simulink model "RobustInvDyn"  (R2024b)
settings: Solver=ode15s  StartTime=0.0  StopTime=10  MinStep=0.0000001
InitFcn:
  | addpath('./../Robot Description/Robot Data Package/meshes/visual/')
  | addpath('./../Dynamics and Kinematics/')
  | 
  | % Controller Design
  | Design;
values from neighbouring files (symbols this model uses):
  alpha = 0.9    [Design.m]
  B = [zeros(n, n); eye(n)]    [Design.m]
  epsilon = 0.01    [Design.m]
  gamma1 = 3.5    [Design.m]
  gamma2 = 1.8    [Design.m]
  gamma3 = 5    [Design.m]
  Kd = 1000    [Design.m]
  Kp = 250000    [Design.m]
  P = lyap(A', Q)    [Design.m]
  qInitDM = [rand(n, 1); zeros(n, 1)]    [Design.m]
settings Model: Creator=Banaan  LastModifiedBy=Asus

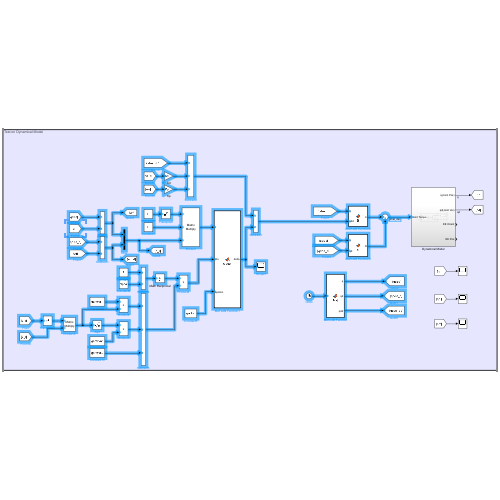
[thumbnail: Simulink's stored preview of the top-level diagram]
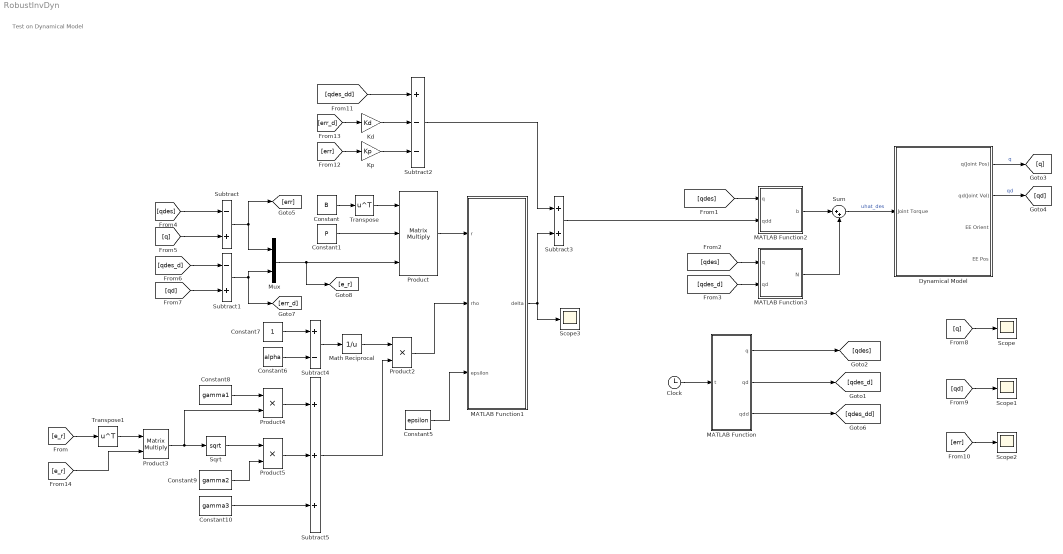
== system RobustInvDyn ==
  note: Test on Dynamical Model
  Clock : Clock
  Constant : Constant  Value=B
  Constant1 : Constant  Value=P
  Constant10 : Constant  Value=gamma3
  Constant5 : Constant  Value=epsilon
  Constant6 : Constant  Value=alpha
  Constant7 : Constant
  Constant8 : Constant  Value=gamma1
  Constant9 : Constant  Value=gamma2
  Dynamical Model : Subsystem
  Kd : Gain  Gain=Kd
  Kp : Gain  Gain=Kp
  MATLAB Function : MATLAB Function  TreatAsAtomicUnit=on
  MATLAB Function1 : MATLAB Function  TreatAsAtomicUnit=on
  MATLAB Function2 : MATLAB Function  TreatAsAtomicUnit=on
  MATLAB Function3 : MATLAB Function  TreatAsAtomicUnit=on
  Math Reciprocal : Math  Operator=reciprocal  SignedPower=on
  Mux : Mux  Inputs=2
  Product : Product  Inputs=3  Multiplication=Matrix(*)
  Product2 : Product
  Product3 : Product  Multiplication=Matrix(*)
  Product4 : Product
  Product5 : Product
  Scope{,1..3} (4 alike) : Scope
  Sqrt : Sqrt
  Subtract : Sum  Inputs=-+
  Subtract1 : Sum  Inputs=-+
  Subtract2 : Sum  Inputs=+--
  Subtract3 : Sum
  Subtract4 : Sum  Inputs=+-
  Subtract5 : Sum  Inputs=+++
  Sum : Sum  Inputs=|++
  Transpose : Math  Operator=transpose
  Transpose1 : Math  Operator=transpose
  wires:
  [qdes] -> MATLAB Function2/1(q)
  [qdes_d] -> MATLAB Function3/2(qd)
  [qdes] -> MATLAB Function3/1(q)
  MATLAB Function2/1(b) -> Sum/1
  MATLAB Function3/1(N) -> Sum/2
  Dynamical Model/1(q(Joint Pos)) -> [q]  "q"
  Dynamical Model/2(qd(Joint Vel)) -> [qd]  "qd"
  [q] -> Scope/1
  [qd] -> Scope1/1
  [err] -> Scope2/1
  MATLAB Function/3(qdd) -> [qdes_dd]
  MATLAB Function/2(qd) -> [qdes_d]
  Clock/1 -> MATLAB Function/1(t)
  MATLAB Function/1(q) -> [qdes]
  [qdes] -> Subtract/1
  [q] -> Subtract/2
  [qdes_d] -> Subtract1/1
  [qd] -> Subtract1/2
  Sum/1 -> Dynamical Model/1(Joint Torque)  "uhat_des"
  [qdes_dd] -> Subtract2/1
  Kd/1 -> Subtract2/2
  Kp/1 -> Subtract2/3
  Subtract/1 -> [err], Mux/1
  Subtract1/1 -> [err_d], Mux/2
  Constant/1 -> Transpose/1
  Transpose/1 -> Product/1
  Constant1/1 -> Product/2
  Mux/1 -> [e_r], Product/3
  Product/1 -> MATLAB Function1/1(r)
  [err] -> Kp/1
  [err_d] -> Kd/1
  MATLAB Function1/1(delta) -> Scope3/1, Subtract3/2
  Subtract2/1 -> Subtract3/1
  Subtract3/1 -> MATLAB Function2/2(qdd)
  Constant5/1 -> MATLAB Function1/3(epsilon)
  Constant7/1 -> Subtract4/1
  Constant6/1 -> Subtract4/2
  Subtract4/1 -> Math Reciprocal/1
  Math Reciprocal/1 -> Product2/1
  Subtract5/1 -> Product2/2
  Product2/1 -> MATLAB Function1/2(rho)
  [e_r] -> Transpose1/1
  Transpose1/1 -> Product3/1
  [e_r] -> Product3/2
  Constant8/1 -> Product4/1
  Product3/1 -> Product4/2, Sqrt/1
  Sqrt/1 -> Product5/1
  Constant9/1 -> Product5/2
  Product4/1 -> Subtract5/1
  Product5/1 -> Subtract5/2
  Constant10/1 -> Subtract5/3

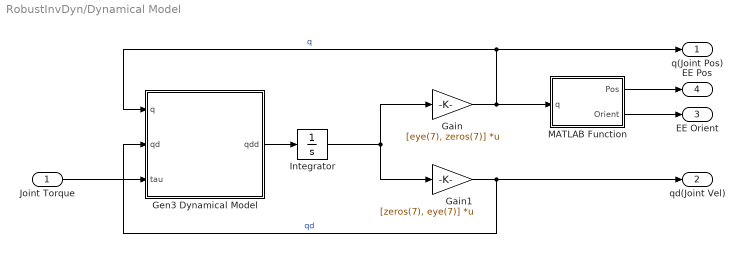
== system RobustInvDyn/Dynamical Model ==
  Joint Torque : Inport
  Gain : Gain  Gain=[eye(7), zeros(7)]  Multiplication=Matrix(K*u)
  Gain1 : Gain  Gain=[zeros(7), eye(7)]  Multiplication=Matrix(K*u)
  Gen3 Dynamical Model : MATLAB Function  TreatAsAtomicUnit=on
  Integrator : Integrator  InitialCondition=qInitDM
  MATLAB Function : MATLAB Function  TreatAsAtomicUnit=on
  q(Joint Pos) : Outport
  qd(Joint Vel) : Outport  Port=2
  EE Orient : Outport  Port=3
  EE Pos : Outport  Port=4
  wires:
  Integrator/1 -> Gain/1, Gain1/1
  Gain/1 -> MATLAB Function/1(q), Gen3 Dynamical Model/1(q), q(Joint Pos)/1  "q"
  Gen3 Dynamical Model/1(qdd) -> Integrator/1
  Gain1/1 -> qd(Joint Vel)/1, Gen3 Dynamical Model/2(qd)  "qd"
  Joint Torque/1 -> Gen3 Dynamical Model/3(tau)
  MATLAB Function/1(Pos) -> EE Pos/1
  MATLAB Function/2(Orient) -> EE Orient/1

== matlab function RobustInvDyn/MATLAB Function2 ==
  data: q input; b output; qdd input
function b = B(q, qdd) %#codegen
    coder.extrinsic('Gen3ODEFun_B');

    tmp = zeros(7, 7);
    tmp = Gen3ODEFun_B(q);

    b = zeros(7, 1);
    b = tmp * qdd;
end

== matlab function RobustInvDyn/Dynamical Model/MATLAB Function ==
  data: q input; Pos output; Orient output
function [Pos, Orient] = FK(q) %#codegen
    coder.extrinsic('Gen3FK');

    tmp = zeros(6, 1);
    tmp = Gen3FK(q);

    Pos    = tmp(1:3, 1);
    Orient = tmp(4:6, 1);      % Order = [Yaw - Pitch - Roll]
end

== matlab function RobustInvDyn/MATLAB Function ==
  data: t input; q output; qd output; qdd output
function [q, qd, qdd] = Traj(t)

    % q   =  ones(7, 1) * sin(t);
    % qd  =  ones(7, 1) * cos(t);
    % qdd = -ones(7, 1) * sin(t);

    q   = ones(7, 1);
    qd  = zeros(7, 1);
    qdd = zeros(7, 1);

end

== matlab function RobustInvDyn/MATLAB Function1 ==
  data: r input; rho input; delta output; epsilon input
function delta = robust(r, rho, epsilon)

    % Robust term
    if r > epsilon
        delta = - rho * r / norm(r, 2);
    else
        delta = - rho * r / epsilon;
    end

end

== matlab function RobustInvDyn/MATLAB Function3 ==
  data: q input; N output; qd input
function N = n(q, qd) %#codegen
    coder.extrinsic('Gen3ODEFun_C');
    coder.extrinsic('Gen3ODEFun_g');

    N = zeros(7, 1);
    C = zeros(7, 7);
    g = zeros(7, 1);
    
    C = Gen3ODEFun_C(q, qd);
    g = Gen3ODEFun_g(q);
    N = C * qd + g;
end

== matlab function RobustInvDyn/Dynamical Model/Gen3 Dynamical Model ==
  data: q input; qdd output; qd input; tau input
function qdd = fcn(q, qd, tau) %#codegen
    coder.extrinsic('Gen3ODEFun');

    qdd = zeros(14, 1);
    qdd = Gen3ODEFun(0, [q; qd], tau);
end
